simulink model "SensingSubsystem"  (R2026a)
settings: Solver=ode15s  StopTime=10  FixedStep=1e-3  MaxStep=1e-6  RelTol=1e-5
model workspace (MAT data in the model file):
  SL_ROS_VariableLengthArrays_MaxSizes.CommonInfo.ArrayTruncateAction = 'EmitWarning'
  SL_ROS_VariableLengthArrays_MaxSizes.MsgTypeMap = containers.Map
  SL_ROS_VariableLengthArrays_MaxSizes.MsgTypeMap.serialization.keys = {'sensor_msgs/Image'}
  SL_ROS_VariableLengthArrays_MaxSizes.MsgTypeMap.serialization.values{1}(1).PropertyName = 'data'
  SL_ROS_VariableLengthArrays_MaxSizes.MsgTypeMap.serialization.values{1}(1).DataType = 'uint8'
  SL_ROS_VariableLengthArrays_MaxSizes.MsgTypeMap.serialization.values{1}(1).MaxLength = 512
  SL_ROS_VariableLengthArrays_MaxSizes.MsgTypeMap.serialization.values{1}(2).PropertyName = 'encoding'
  SL_ROS_VariableLengthArrays_MaxSizes.MsgTypeMap.serialization.values{1}(2).DataType = 'uint8'
  SL_ROS_VariableLengthArrays_MaxSizes.MsgTypeMap.serialization.values{1}(2).MaxLength = 128
  SL_ROS_VariableLengthArrays_MaxSizes.MsgTypeMap.serialization.uniformity = 0
  SL_ROS_VariableLengthArrays_MaxSizes.MsgTypeMap.serialization.keyType = 'char'
  SL_ROS_VariableLengthArrays_MaxSizes.MsgTypeMap.serialization.valueType = 'any'
undefined symbols (not defined in the file or in its folder): AS7341_8Channel, BPW34_Photodiode, DS18B20_Temperature, MS5837_Pressure, sandy_sensors
libraries: fl_lib x32, nesl_utility x22, ee_lib x6, ros2lib x4
(part 1 of 2)
settings Model: Creator=skips  LastModifiedBy=skips
settings HardwareCC: ProdBitPerLong=64.0  ProdHWDeviceType=Intel->x86-64 (Linux 64)  UseEmbeddedCoderFeatures=off
settings RTWCC: SystemTargetFile=ert.tlc  HardwareBoard=Robot Operating System 2 (ROS 2)  TLCOptions="-aInlineSetEventsForThisBaseRateFcn=TLC_FALSE -aSuppressMultiTaskScheduler=TLC_FALSE  -aRateBasedStepFcn=0"  Toolchain=Colcon Tools  TargetLang=C++  Description=Embedded Coder
settings ERTTargetCC: ExtModeTransport=2.0  ExtModeAutomaticAllocSize=off  RootIOFormat=Structure reference  CodeInterfacePackaging=C++ class  SupportNonInlinedSFcns=on

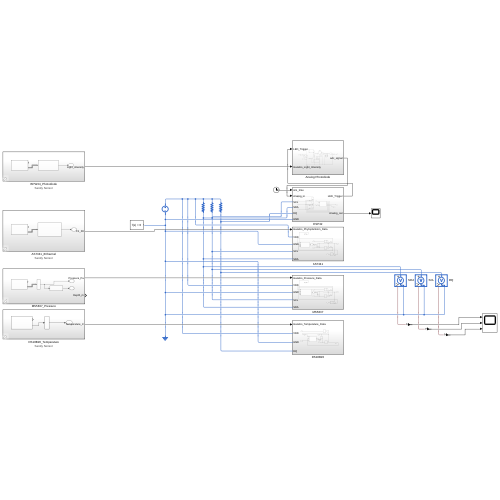
[thumbnail: Simulink's stored preview of the top-level diagram]
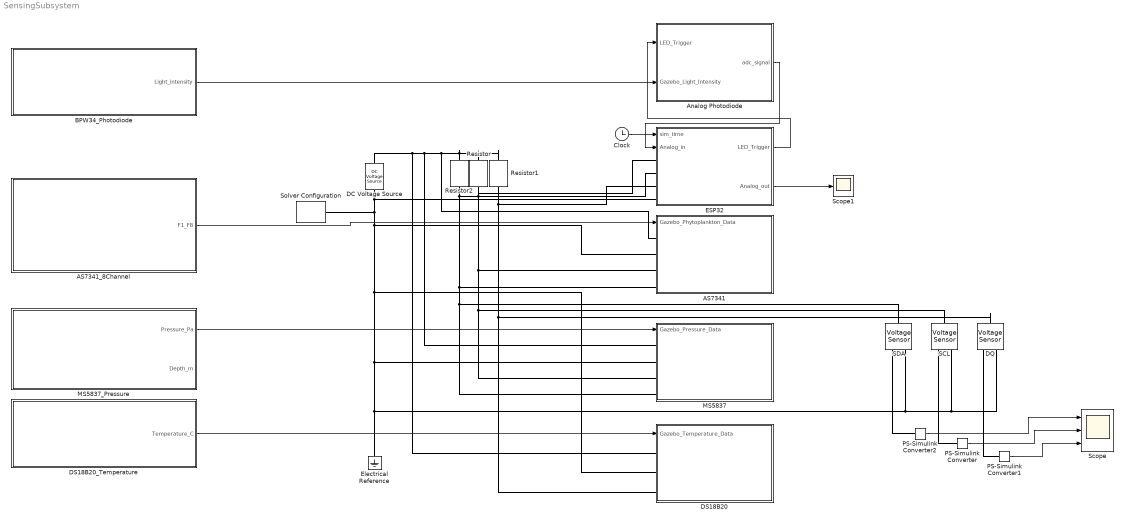
== system SensingSubsystem ==
  AS7341 : Subsystem
  AS7341_8Channel : Subsystem  Description=AS7341 8-channel proxy. Subscribes to /sandy/as7341_down (sensor_msgs/Image, 8x8 RGB from Gazebo) and synthesises 8 spectral channels F1..F8 (415, 445, 480, 515, 555, 590, 630, 680 nm). Output is uint16(1x8), matching the AS7341 16-bit ADC range. NOTE: This is a synthesis from broadband RGB. Useful for testing detection logic and data pipelines; not physically accurate for spectral retrieval algorithms.  AncestorBlock=sandy_sensors/AS7341_8Channel
      settings: AttributesFormatString=Sandy Sensor
  Analog Photodiode : Subsystem
  BPW34_Photodiode : Subsystem  Description=BPW34 photodiode proxy. Subscribes to /sandy/photodiode_side (sensor_msgs/Image, 4x4 RGB from Gazebo) and outputs a scalar irradiance in [0, 1]. Multiply by your photocurrent scale factor (e.g. 5e-7 A) before feeding into the TIA.  AncestorBlock=sandy_sensors/BPW34_Photodiode
      settings: AttributesFormatString=Sandy Sensor
  Clock : Clock
  DC Voltage Source : ee_lib/Additional Components/SPICE Sources/DC Voltage Source  DC=3.3 V
  DQ : fl_lib/Electrical/Electrical Sensors/Voltage Sensor
  DS18B20 : Subsystem
  DS18B20_Temperature : Subsystem  Description=DS18B20 temperature proxy. Subscribes to /sandy/temperature (sensor_msgs/Temperature, published by the helper node from the Antarctic depth profile OR a manual slider). Outputs scalar T in C.  AncestorBlock=sandy_sensors/DS18B20_Temperature
      settings: AttributesFormatString=Sandy Sensor
  ESP32 : Subsystem
  Electrical Reference : fl_lib/Electrical/Electrical Elements/Electrical Reference
  MS5837 : Subsystem
  MS5837_Pressure : Subsystem  Description=MS5837-30BA proxy. Subscribes to /sandy/pressure (sensor_msgs/FluidPressure, computed from buoy Z by the helper node). Outputs absolute pressure in Pa AND depth in m (depth = (P - 101325) / (1028 * 9.80665)).  AncestorBlock=sandy_sensors/MS5837_Pressure
      settings: AttributesFormatString=Sandy Sensor
  PS-Simulink Converter : nesl_utility/PS-Simulink Converter  PhysicalDomain=network_engine_domain  SubClassName=ps_output  LeftPortType=input  RightPortType=output  PseudoPeriodic=off  Frequencies=[]  VectorFormat=inherit  Unit=inherit  AffineConversion=off
  PS-Simulink Converter1 : nesl_utility/PS-Simulink Converter  PhysicalDomain=network_engine_domain  SubClassName=ps_output  LeftPortType=input  RightPortType=output  PseudoPeriodic=off  Frequencies=[]  VectorFormat=inherit  Unit=inherit  AffineConversion=off
  PS-Simulink Converter2 : nesl_utility/PS-Simulink Converter  PhysicalDomain=network_engine_domain  SubClassName=ps_output  LeftPortType=input  RightPortType=output  PseudoPeriodic=off  Frequencies=[]  VectorFormat=inherit  Unit=inherit  AffineConversion=off
  Resistor : fl_lib/Electrical/Electrical Elements/Resistor  R=4700 Ohm  i_specify=off  i_priority=None  i=0 A  i_nominal_specify=off  i_nominal_value=1  i_nominal_unit=A  v_specify=off  v_priority=None  v=0 V  v_nominal_specify=off  v_nominal_value=1  v_nominal_unit=V
  Resistor1 : fl_lib/Electrical/Electrical Elements/Resistor  R=4700 Ohm  i_specify=off  i_priority=None  i=0 A  i_nominal_specify=off  i_nominal_value=1  i_nominal_unit=A  v_specify=off  v_priority=None  v=0 V  v_nominal_specify=off  v_nominal_value=1  v_nominal_unit=V
  Resistor2 : fl_lib/Electrical/Electrical Elements/Resistor  R=4700 Ohm  i_specify=off  i_priority=None  i=0 A  i_nominal_specify=off  i_nominal_value=1  i_nominal_unit=A  v_specify=off  v_priority=None  v=0 V  v_nominal_specify=off  v_nominal_value=1  v_nominal_unit=V
  SCL : fl_lib/Electrical/Electrical Sensors/Voltage Sensor
  SDA : fl_lib/Electrical/Electrical Sensors/Voltage Sensor
  Scope : Scope  NumInputPorts=3
      settings: ActiveDisplayYMinimum=3.1434378707500259  ActiveDisplayYMaximum=3.3880168227126775
  Scope1 : Scope
      settings: ActiveDisplayYMinimum=-121086.7377727352  ActiveDisplayYMaximum=114154.80125551928
  Solver Configuration : nesl_utility/Solver Configuration  PhysicalDomain=network_engine_domain  SubClassName=solver  LeftPortType=input  RightPortType=generic  Tones=[]  Harmonics=[]  SimulateNoise=off  Profile=off  UseLocalSampling=off  EnableSwitchedLinearOptims=on  FrequencyDomain=off  UseCCode=off  RelTol=0.001  AbsTol=0.001  MinStep=1e-09  ToWorkspace=off  RevertToSquareIcSolve=off  NumHomotopyIterations=100  PhasorMode=off  PhasorModeNumHarmonics=1  ConsistencySolver=NEWTON_XTOL_AFTER_FTOL  CanonicalOrdering=CANONICAL  OptimizeIntermediates=OPTIMIZED  IndexReductionMethod=DerivativeReplacement  DoDC=off  ResidualTolerance=1e-09  ConsistencyTolSource=GLOBAL  ConsistencyAbsTol=0.001  ConsistencyRelTol=0.001  ConsistencyTolFactor=0.001  UseLocalSolver=off  LocalSolverChoice=NE_BACKWARD_EULER_ADVANCER  ResolveIndetEquations=on  FunctionEvalNumThread=1  LocalSolverSampleTime=0.001  DoFixedCost=off  MaxNonlinIter=3  MaxModeIter=2  ComputeImpulses=off  ImpulseIterations=2  LinearAlgebra=auto  LinearAlgebraNumThread=0  EquationFormulation=NE_TIME_EF  DelaysMemoryBudget=1024  AutomaticFiltering=on  FilteringTimeConstant=0.001  PartitionStorageMethod=AS_NEEDED  PartitionMemoryBudget=1024  PartitionMethod=ROBUST  MultibodyUseLocalSolver=off  MultibodyLocalSolverChoice=ODE1  MultibodyLocalSolverSampleTime=0.001
  wires:
  Clock/1 -> ESP32/1(sim_time)
  PS-Simulink Converter2/1 -> Scope/1
  PS-Simulink Converter/1 -> Scope/2
  PS-Simulink Converter1/1 -> Scope/3
  AS7341_8Channel/1(F1_F8) -> AS7341/1(Gazebo_Phytoplankton_Data)
  DS18B20_Temperature/1(Temperature_C) -> DS18B20/1(Gazebo_Temperature_Data)
  Analog Photodiode/1(adc_signal) -> ESP32/2(Analog_in)
  ESP32/1(LED_Trigger) -> Analog Photodiode/1(LED_Trigger)
  ESP32/2(Analog_out) -> Scope1/1
  BPW34_Photodiode/1(Light_intensity) -> Analog Photodiode/2(Gazebo_Light_Intensity)
  MS5837_Pressure/1(Pressure_Pa) -> MS5837/1(Gazebo_Pressure_Data)
  connections:
  Electrical Reference/LConn1 -- SDA/RConn2 -- DQ/RConn2 -- SCL/RConn2 -- ESP32/LConn4 -- DC Voltage Source/RConn1 -- Solver Configuration/RConn1 -- AS7341/LConn2 -- DS18B20/LConn2 -- MS5837/LConn2
  Resistor/LConn1 -- AS7341/LConn1 -- MS5837/LConn1 -- DS18B20/LConn1 -- DC Voltage Source/LConn1 -- Resistor2/LConn1 -- Resistor1/LConn1
  Resistor1/RConn1 -- DQ/LConn1 -- DS18B20/LConn3 -- ESP32/LConn3
  Resistor/RConn1 -- SCL/LConn1 -- MS5837/LConn3 -- AS7341/LConn3 -- ESP32/LConn1
  Resistor2/RConn1 -- ESP32/LConn2 -- SDA/LConn1 -- MS5837/LConn4 -- AS7341/LConn4
  SDA/RConn1 -- PS-Simulink Converter2/LConn1
  SCL/RConn1 -- PS-Simulink Converter/LConn1
  DQ/RConn1 -- PS-Simulink Converter1/LConn1

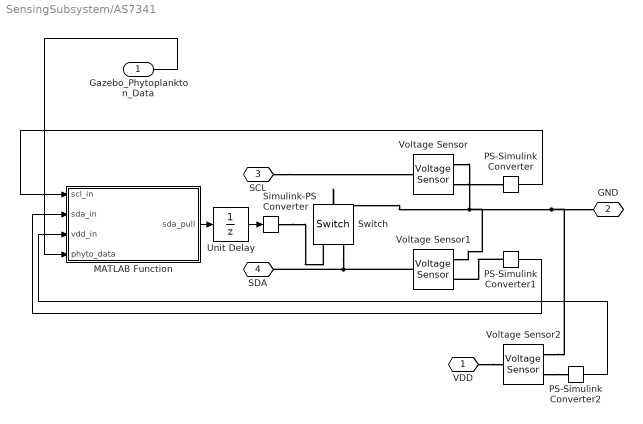
== system SensingSubsystem/AS7341 ==
  Gazebo_Phytoplankton_Data : Inport
  MATLAB Function : MATLAB Function  TreatAsAtomicUnit=on  SystemSampleTime=1e-3
  PS-Simulink Converter : nesl_utility/PS-Simulink Converter  PhysicalDomain=network_engine_domain  SubClassName=ps_output  LeftPortType=input  RightPortType=output  PseudoPeriodic=off  Frequencies=[]  VectorFormat=inherit  Unit=inherit  AffineConversion=off
  PS-Simulink Converter1 : nesl_utility/PS-Simulink Converter  PhysicalDomain=network_engine_domain  SubClassName=ps_output  LeftPortType=input  RightPortType=output  PseudoPeriodic=off  Frequencies=[]  VectorFormat=inherit  Unit=inherit  AffineConversion=off
  PS-Simulink Converter2 : nesl_utility/PS-Simulink Converter  PhysicalDomain=network_engine_domain  SubClassName=ps_output  LeftPortType=input  RightPortType=output  PseudoPeriodic=off  Frequencies=[]  VectorFormat=inherit  Unit=inherit  AffineConversion=off
  Simulink-PS Converter : nesl_utility/Simulink-PS Converter  PhysicalDomain=network_engine_domain  SubClassName=ps_input  LeftPortType=input  RightPortType=output  PseudoPeriodic=off  Frequencies=[]  NoiseDistribution=none  NoiseParameters=[]  Unit=1  AffineConversion=off  FilteringAndDerivatives=provide  SimscapeFilterOrder=1  InputFilterTimeConstant=0.001  UdotUserProvided=0
  Switch : fl_lib/Electrical/Electrical Elements/Switch  R_closed=0.01 Ohm  G_open=1e-8 1/Ohm  Threshold=0.5  i_specify=off  i_priority=None  i=0 A  i_nominal_specify=off  i_nominal_value=1  i_nominal_unit=A  v_specify=off  v_priority=None  v=0 V  v_nominal_specify=off  v_nominal_value=1  v_nominal_unit=V
  Unit Delay : UnitDelay  SampleTime=-1
  Voltage Sensor : fl_lib/Electrical/Electrical Sensors/Voltage Sensor
  Voltage Sensor1 : fl_lib/Electrical/Electrical Sensors/Voltage Sensor
  Voltage Sensor2 : fl_lib/Electrical/Electrical Sensors/Voltage Sensor
  VDD : PMIOPort  Side=Left
  GND : PMIOPort  Port=2  Side=Left
  SCL : PMIOPort  Port=3  Side=Left
  SDA : PMIOPort  Port=4  Side=Left
  wires:
  PS-Simulink Converter1/1 -> MATLAB Function/2(sda_in)
  PS-Simulink Converter/1 -> MATLAB Function/1(scl_in)
  PS-Simulink Converter2/1 -> MATLAB Function/3(vdd_in)
  Gazebo_Phytoplankton_Data/1 -> MATLAB Function/4(phyto_data)
  Unit Delay/1 -> Simulink-PS Converter/1
  MATLAB Function/1(sda_pull) -> Unit Delay/1
  connections:
  SCL/RConn1 -- Voltage Sensor/LConn1
  Voltage Sensor/RConn2 -- Voltage Sensor1/RConn2 -- Voltage Sensor2/RConn2 -- GND/RConn1 -- Switch/LConn1
  Voltage Sensor1/LConn1 -- Switch/RConn2 -- SDA/RConn1
  Voltage Sensor/RConn1 -- PS-Simulink Converter/LConn1
  PS-Simulink Converter1/LConn1 -- Voltage Sensor1/RConn1
  Simulink-PS Converter/RConn1 -- Switch/RConn1
  VDD/RConn1 -- Voltage Sensor2/LConn1
  Voltage Sensor2/RConn1 -- PS-Simulink Converter2/LConn1

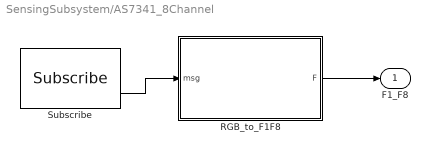
== system SensingSubsystem/AS7341_8Channel ==
  RGB_to_F1F8 : MATLAB Function  TreatAsAtomicUnit=on
  Subscribe : ros2lib/Subscribe  topicSource=Specify your own  topic=/sandy/as7341_down  messageType=sensor_msgs/Image  sampleTime=0.1  QOSHistory=Keep last  QOSDepth=5  QOSReliability=Best effort  QOSDurability=Volatile  QOSDeadline=Inf  QOSLifespan=Inf  QOSLiveliness=Automatic  QOSLeaseDuration=Inf  QOSAvoidROSNamespaceConventions=off
  F1_F8 : Outport
  wires:
  RGB_to_F1F8/1(F) -> F1_F8/1
  Subscribe/2 -> RGB_to_F1F8/1(msg)

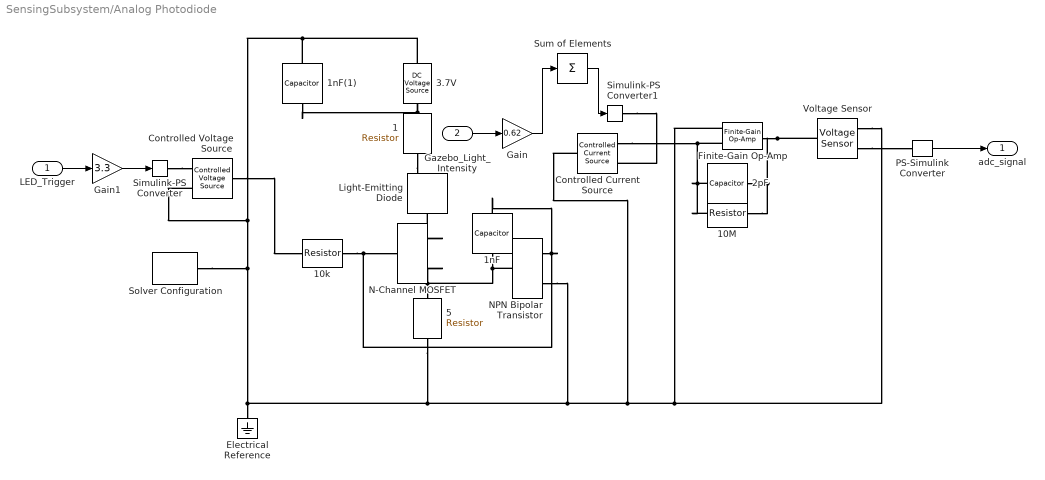
== system SensingSubsystem/Analog Photodiode ==
  LED_Trigger : Inport
  Gazebo_Light_Intensity : Inport  Port=2
  1 : fl_lib/Electrical/Electrical Elements/Resistor  R=1 Ohm  i_specify=off  i_priority=None  i=0 A  i_nominal_specify=off  i_nominal_value=1  i_nominal_unit=A  v_specify=off  v_priority=None  v=0 V  v_nominal_specify=off  v_nominal_value=1  v_nominal_unit=V
  10M : fl_lib/Electrical/Electrical Elements/Resistor  R=10 MOhm  i_specify=off  i_priority=None  i=0 A  i_nominal_specify=off  i_nominal_value=1  i_nominal_unit=A  v_specify=off  v_priority=None  v=0 V  v_nominal_specify=off  v_nominal_value=1  v_nominal_unit=V
  10k : fl_lib/Electrical/Electrical Elements/Resistor  R=10000 Ohm  i_specify=off  i_priority=None  i=0 A  i_nominal_specify=off  i_nominal_value=1  i_nominal_unit=A  v_specify=off  v_priority=None  v=0 V  v_nominal_specify=off  v_nominal_value=1  v_nominal_unit=V
  1nF : fl_lib/Electrical/Electrical Elements/Capacitor  c=2e-9 F  r=1e-6 Ohm  g=0 1/Ohm  i_specify=off  i_priority=None  i=0 A  i_nominal_specify=off  i_nominal_value=1  i_nominal_unit=A  v_specify=off  v_priority=None  v=0 V  v_nominal_specify=off  v_nominal_value=1  v_nominal_unit=V  vc_specify=off  vc_priority=High  vc=0 V  vc_nominal_specify=off  vc_nominal_value=1  vc_nominal_unit=V
  1nF(1) : fl_lib/Electrical/Electrical Elements/Capacitor  c=1 nF  r=1e-6 Ohm  g=0 1/Ohm  i_specify=off  i_priority=None  i=0 A  i_nominal_specify=off  i_nominal_value=1  i_nominal_unit=A  v_specify=off  v_priority=None  v=0 V  v_nominal_specify=off  v_nominal_value=1  v_nominal_unit=V  vc_specify=off  vc_priority=High  vc=0 V  vc_nominal_specify=off  vc_nominal_value=1  vc_nominal_unit=V
  2pF : fl_lib/Electrical/Electrical Elements/Capacitor  c=2 pF  r=1e-6 Ohm  g=0 1/Ohm  i_specify=off  i_priority=None  i=0 A  i_nominal_specify=off  i_nominal_value=1  i_nominal_unit=A  v_specify=off  v_priority=None  v=0 V  v_nominal_specify=off  v_nominal_value=1  v_nominal_unit=V  vc_specify=off  vc_priority=High  vc=0 V  vc_nominal_specify=off  vc_nominal_value=1  vc_nominal_unit=V
  3.7V : ee_lib/Additional Components/SPICE Sources/DC Voltage Source  DC=3.7 V
  5 : fl_lib/Electrical/Electrical Elements/Resistor  R=5 Ohm  i_specify=off  i_priority=None  i=0 A  i_nominal_specify=off  i_nominal_value=1  i_nominal_unit=A  v_specify=off  v_priority=None  v=0 V  v_nominal_specify=off  v_nominal_value=1  v_nominal_unit=V
  Controlled Current Source : fl_lib/Electrical/Electrical Sources/Controlled Current Source
  Controlled Voltage Source : fl_lib/Electrical/Electrical Sources/Controlled Voltage Source
  Electrical Reference : fl_lib/Electrical/Electrical Elements/Electrical Reference
  Finite-Gain Op-Amp : ee_lib/Integrated Circuits/Finite-Gain Op-Amp  A=1e5  Rin=1e12 Ohm  Rout=10 Ohm  Vmin=0.02 V  Vmax=3.3 V  noise_mode=ee.enum.mode.enabled  v_noise=30e-9 V/Hz^(1/2)  noise_prm=ee.enum.ic.noiseParameterization.same  i_noise=0.6e-15 A/Hz^(1/2)  ip_noise=0.5e-12 A/Hz^(1/2)  in_noise=0.5e-12 A/Hz^(1/2)  sample_time=1e-3 s  repeatability=ee.enum.ic.repeatability.notRepeatable  auto_seed_v=3890346746  auto_seed_ip=545404223  auto_seed_in=3922919431  user_seed_v=0  user_seed_ip=0  user_seed_in=0
  Gain : Gain  Gain=0.62  OutDataTypeStr=Inherit: Same as input
  Gain1 : Gain  Gain=3.3
  Light-Emitting Diode : ee_lib/Sensors & Transducers/Light-Emitting Diode  Gain=0.005 W/A  prmExp=ee.enum.diode.led.useTwo  I12=[.0017, .003] A  V12=[.9, 1.05] V  IS=5e-5 A  ec=10  RS=0.1 Ohm  Tmeas=25 degC  C_param=ee.enum.diode.capParam.fixed  CJ=20 pF  CJ0=20 pF  Vvec=[.1, 10, 100] V  Cvec=[15, 10, 2] pF  VJ=1 V  Mgrad=0.5  FC=0.5  T_param=ee.enum.diode.temperatureParam.off  Tdevice=25 degC  IS_T2=1.8e-4 A  I1_T2=0.0034 A  V1_T2=1.05 V  Tmeas2=125 degC  EG_param=ee.enum.diode.egapParam.material_si  EG=1.11 eV  XTI_param=ee.enum.diode.xtiParam.pn  XTI=3  i_specify=off  i_priority=None  i=0 A  i_nominal_specify=off  i_nominal_value=1  i_nominal_unit=A  v_specify=off  v_priority=None  v=0 V  v_nominal_specify=off  v_nominal_value=1  v_nominal_unit=V  v_capacitor_specify=off  v_capacitor_priority=None  v_capacitor=0 V  v_capacitor_nominal_specify=off  v_capacitor_nominal_value=1  v_capacitor_nominal_unit=V  Qj_specify=off  Qj_priority=High  Qj=0 C  Qj_nominal_specify=off  Qj_nominal_value=1  Qj_nominal_unit=C  thermal_network_parameterization=ee.enum.thermalNetworkTopology.junctionCase  Rth=[0, 10] K/W  Rth_Cauer=[1, 3, 10] K/W  Rth_Foster=[.08, .14, .22, .16] K/W  thermal_mass_parameterization=ee.enum.thermalNetwork.timeconstant  thermal_mass=[0, 1] J/K  thermal_mass_Cauer=[1.5, 2, 3] J/K  thermal_mass_Foster=[.001, .005, .05, .5] J/K  thermal_time_constant=[0, 10] s  thermal_time_constant_Cauer=[1, 3, 10] s  thermal_time_constant_Foster=[7e-05, .0007, .01, .08] s  thermal_mass_initial_temperatures=[25, 25] degC  thermal_mass_initial_temperatures_Cauer=[25, 25, 25] degC  steadyState_Foster=simscape.enum.onoff.on  Tvec_initial_Foster=[25, 25, 25, 25] degC
  N-Channel MOSFET : ee_lib/Semiconductors & Converters/N-Channel MOSFET  paramTerminal=ee.enum.mosfet.numberOfTerminals.three  parameterization=ee.enum.mosfet.parameterization.datasheet  Beta=5.0 A/V^2  Rds=0.035 Ohm  Id=16 A  Vgs=5 V  Vth=2.1 V  Vth0=1.7 V  lam=0 1/V  gamma_vth=0.5 V^(1/2)  phib=0.5 V  Vth1=1.9071 V  Vbs1=-1 V  Vth2=2.066 V  Vbs2=-2 V  Tmeas=0 degC  Vgs_vec=[-1, -.5, 2, 3, 4, 5] V  Vds_vec=[0, 2, 4, 8, 12, 16, 20] V  Vbs_vec=[0, -4, -6, -12] V  T_vec=[25, 125] degC  Vth_vec=[.4, 1.2, 1.4, 1.45] V  Vth_mat=[.4, .35; 1.2, 1.15; 1.4, 1.35; 1.45, 1.4] V  Ids_mat=[0, 0, 0, 0, 0, 0, 0; 0, 0, 0, 0, 0, 0, 0; 0, .003, .0038, .0043, .0046, .0048, .0049; 0, .0055, .008, .009, .0095, .01, .0101; 0, .0115, .016, .018, .019, .0195, .02; 0, .0152, .0225, .0265, .028, .0295, .03] A  Ids_mat0=[0, 0, 0, 0, 0, 0, 0; 0, 0, 0, 0, 0, 0, 0; 0, .003, .0038, .0043, .0046, .0048, .0049; 0, .0055, .008, .009, .0095, .01, .0101; 0, .0115, .016, .018, .019, .0195, .02; 0, .0152, .0225, .0265, .028, .0295, .03] A  Ids_mat_3D=zeros(6, 7, 2) A  Ids_mat_3D0=zeros(6, 7, 2) A  IV_table_symmetry=ee.enum.mosfet.symmetricNIV.no  RS=0.0001 Ohm  RD=0.01 Ohm  RB=0.001 Ohm  LeadRs=0 Ohm  LeadRd=0 Ohm  LeadRg=0 Ohm  LeadRb=0 Ohm  LS=0 nH  LD=0 nH  LG=0 nH  LB=0 nH  C_param=ee.enum.mosfet.capacitanceParam.fixedciss  C_GS=270 pF  C_GD=80 pF  C_GB=0 pF  C_DS=0 pF  C_iss=1000 pF  C_rss=120 pF  C_oss=0 pF  C_iss_vec=[720, 700, 590, 470, 390, 310] pF  C_rss_vec=[450, 400, 300, 190, 95, 55] pF  C_oss_vec=[900, 810, 690, 420, 270, 170] pF  C_GS_vec=[270, 300, 290, 280, 295, 255] pF  C_GD_vec=[450, 400, 300, 190, 95, 55] pF  C_GB_vec=[270, 300, 290, 280, 295, 255] pF  C_Vgs_vec=0 V  C_DS_vec=[450, 410, 390, 230, 175, 115] pF  C_Vds_vec=[.1, .3, 1, 3, 10, 30] V  V_GS_for_cap_data=0 V  charge_linearity_param=ee.enum.mosfet.cgdLinearity.constant  C_OX=200 pF  V_C_OX=-0.5 V  charge_linearity_param_vgb=ee.enum.mosfet.cgbLinearity.instantly  charge_linearity_param_with_vgb=ee.enum.mosfet.cgbLinearityWithSeparateCgb.instantly  Di_param=ee.enum.mosfet.diodeParam.no  IsDiode=1e-12 A  Vbi=0.6 V  n=1  Cj0Diode=0 pF  TT=50e-9 s  Tmeas_dio=25 degC  TableTypeNoT=ee.enum.mosfet.tableType.IfMat  TableType=ee.enum.diode.tableType.IfMat  IfVec=[.07, .12, .19, 1.75, 4.24, 7.32, 11.2] A  IfMat=[.07, .12, .19, 1.75, 4.24, 7.32, 11.2; .16, .3, .72, 2.14, 4.02, 6.35, 9.12] A  VfVecV=[.9, 1.15, 1.25, 1.5, 1.75, 2.17, 2.6, 2.85] V  VfMatV=[.9, 1.15, 1.25, 1.5, 1.75, 2.17, 2.6, 2.85; .58, .68, .75, 1.1, 1.38, 1.77, 2.27, 2.7] V  TjVec=[25, 125] degC  VfVec=[.5, .7, .9, 1.3, 1.7, 2.1, 2.5] V  IfVecV=[.1, .2, .5, 1, 2, 4, 7, 10] A  diode_Goff=1e-12 1/Ohm  prmDatasheet=ee.enum.temperatureParameterization.none  prmEquCoeff=ee.enum.temperatureParameterization.none  dVth_dT=-6 mV/K  dVth0_dT=-6 mV/K  Rds_T2=0.037 Ohm  BEXDatasheet=-1.5  BEXEquCoeff=-1.5  etaisDatasheet=3  etaisEquCoeff=3  Tmeas2=125 degC  etaisTabulated=3  TdeviceDatasheet=25 degC  TdeviceEquCoeff=25 degC  TdeviceTabulated=25 degC  i_g_specify=off  i_g_priority=None  i_g=0 A  i_g_nominal_specify=off  i_g_nominal_value=1  i_g_nominal_unit=A  i_d_specify=off  i_d_priority=None  i_d=0 A  i_d_nominal_specify=off  i_d_nominal_value=1  i_d_nominal_unit=A  i_b_specify=off  i_b_priority=None  i_b=0 A  i_b_nominal_specify=off  i_b_nominal_value=1  i_b_nominal_unit=A  voltage_gs_specify=off  voltage_gs_priority=None  voltage_gs=0 V  voltage_gs_nominal_specify=off  voltage_gs_nominal_value=1  voltage_gs_nominal_unit=V  voltage_ds_specify=off  voltage_ds_priority=None  voltage_ds=0 V  voltage_ds_nominal_specify=off  voltage_ds_nominal_value=1  voltage_ds_nominal_unit=V  voltage_bs_specify=off  voltage_bs_priority=None  voltage_bs=0 V  voltage_bs_nominal_specify=off  voltage_bs_nominal_value=1  voltage_bs_nominal_unit=V  v_Cgs_specify=off  v_Cgs_priority=High  v_Cgs=0 V  v_Cgs_nominal_specify=off  v_Cgs_nominal_value=1  v_Cgs_nominal_unit=V  v_Cds_specify=off  v_Cds_priority=High  v_Cds=0 V  v_Cds_nominal_specify=off  v_Cds_nominal_value=1  v_Cds_nominal_unit=V  v_Cbs_specify=off  v_Cbs_priority=High  v_Cbs=0 V  v_Cbs_nominal_specify=off  v_Cbs_nominal_value=1  v_Cbs_nominal_unit=V  thermal_network_parameterization=ee.enum.thermalNetworkTopology.junctionCase  Rth=[0, 10] K/W  Rth_Cauer=[1, 3, 10] K/W  Rth_Foster=[.08, .14, .22, .16] K/W  thermal_mass_parameterization=ee.enum.thermalNetwork.timeconstant  thermal_mass=[0, 1] J/K  thermal_mass_Cauer=[.1, .3, 1] J/K  thermal_mass_Foster=[.001, .005, .05, .5] J/K  thermal_time_constant=[0, 10] s  thermal_time_constant_Cauer=[1, 3, 10] s  thermal_time_constant_Foster=[7e-05, .0007, .01, .08] s  thermal_mass_initial_temperatures=[25, 25] degC  thermal_mass_initial_temperatures_Cauer=[25, 25, 25] degC  Tvec_initial_Foster=[25, 25, 25, 25] degC  betaref=18 A/V^2  Vfbref=-1.1 V  gamma=3.5 V^(1/2)  phib2ref=1 V  thesatref=0.4 1/V  alpha=0  Vp=5e-2 V  thesrref=0 1/V  m=8  Tref=25 degC  Rsref=2e-3 Ohm  Rdref=0.17 Ohm  Rgref=8.4 Ohm  Rbref=2e-3 Ohm  Cox=1500 pF  Cgso=100 pF  Cgdo=14 pF  Isref=5.2e-13 A  Cj0=480 pF  Tprm=ee.enum.temperatureParameterization.none  etabet=1.3  Stvfb=5e-4 V/K  Stphib=-8.5e-4 V/K  etasat=1.04  etasr=0.65  etar=0.95  etais=3  Tsim=25 degC  Ig_specify=off  Ig_priority=None  Ig=0 A  Ig_nominal_specify=off  Ig_nominal_value=1  Ig_nominal_unit=nA  Ids_specify=off  Ids_priority=None  Ids=0 A  Ids_nominal_specify=off  Ids_nominal_value=1  Ids_nominal_unit=A  Ib_specify=off  Ib_priority=None  Ib=0 A  Ib_nominal_specify=off  Ib_nominal_value=1  Ib_nominal_unit=uA  V_gs_specify=off  V_gs_priority=None  V_gs=0 V  V_gs_nominal_specify=off  V_gs_nominal_value=1  V_gs_nominal_unit=V  V_ds_specify=off  V_ds_priority=None  V_ds=0 V  V_ds_nominal_specify=off  V_ds_nominal_value=1  V_ds_nominal_unit=V  V_bs_specify=off  V_bs_priority=None  V_bs=0 V  V_bs_nominal_specify=off  V_bs_nominal_value=1  V_bs_nominal_unit=V  QGoverCox_specify=off  QGoverCox_priority=None  QGoverCox=0 V  QGoverCox_nominal_specify=off  QGoverCox_nominal_value=1  QGoverCox_nominal_unit=V  QDoverCox_specify=off  QDoverCox_priority=None  QDoverCox=0 V  QDoverCox_nominal_specify=off  QDoverCox_nominal_value=1  QDoverCox_nominal_unit=V  QBoverCox_specify=off  QBoverCox_priority=None  QBoverCox=0 V  QBoverCox_nominal_specify=off  QBoverCox_nominal_value=1  QBoverCox_nominal_unit=V  T0=[25, 25] degC  T0_Cauer=[25, 25, 25] degC
  NPN Bipolar Transistor : ee_lib/Semiconductors & Converters/NPN Bipolar Transistor  parameterization=1  BF=100  IS=1e-14 A  VAF=200 V  hfe=300  hoe=50e-6 1/Ohm  Ic_h=1 mA  Vce_h=5 V  V1=0.65 V  I1=0.5 mA  BR=1  Tmeas=0 degC  RC=0.01 Ohm  RE=1e-4 Ohm  RB=1 Ohm  C_BC=5 pF  C_BE=5 pF  TF=0 us  TR=0 us  prmDatasheet=1  prmEquCoeff=1  hfe_T2=125  XTB=0  V1_T2=0.45 V  I1_T2=0.5 mA  Tmeas2=125 degC  EG=1.11 eV  XTI=3  TdeviceDatasheet=25 degC  TdeviceEquCoeff=25 degC  ec=1  ib_specify=off  ib_priority=None  ib=0 A  ib_nominal_specify=off  ib_nominal_value=1  ib_nominal_unit=A  ic_specify=off  ic_priority=None  ic=0 A  ic_nominal_specify=off  ic_nominal_value=1  ic_nominal_unit=A  vce_specify=off  vce_priority=None  vce=0 V  vce_nominal_specify=off  vce_nominal_value=1  vce_nominal_unit=V  vbe_specify=off  vbe_priority=None  vbe=0 V  vbe_nominal_specify=off  vbe_nominal_value=1  vbe_nominal_unit=V  Qbc_specify=off  Qbc_priority=High  Qbc=0 C  Qbc_nominal_specify=off  Qbc_nominal_value=1  Qbc_nominal_unit=uC  Qbe_specify=off  Qbe_priority=High  Qbe=0 C  Qbe_nominal_specify=off  Qbe_nominal_value=1  Qbe_nominal_unit=uC  thermal_network_parameterization=ee.enum.thermalNetworkTopology.junctionCase  Rth=[0, 10] K/W  Rth_Cauer=[1, 3, 10] K/W  Rth_Foster=[.08, .14, .22, .16] K/W  thermal_mass_parameterization=ee.enum.thermalNetwork.timeconstant  thermal_mass=[0, 1] J/K  thermal_mass_Cauer=[.1, .3, 1] J/K  thermal_mass_Foster=[.001, .005, .05, .5] J/K  thermal_time_constant=[0, 10] s  thermal_time_constant_Cauer=[1, 3, 10] s  thermal_time_constant_Foster=[7e-05, .0007, .01, .08] s  thermal_mass_initial_temperatures=[25, 25] degC  thermal_mass_initial_temperatures_Cauer=[25, 25, 25] degC  Tvec_initial_Foster=[25, 25, 25, 25] degC
  PS-Simulink Converter : nesl_utility/PS-Simulink Converter  PhysicalDomain=network_engine_domain  SubClassName=ps_output  LeftPortType=input  RightPortType=output  PseudoPeriodic=off  Frequencies=[]  VectorFormat=inherit  Unit=V  AffineConversion=off
  Simulink-PS Converter : nesl_utility/Simulink-PS Converter  PhysicalDomain=network_engine_domain  SubClassName=ps_input  LeftPortType=input  RightPortType=output  PseudoPeriodic=off  Frequencies=[]  NoiseDistribution=none  NoiseParameters=[]  Unit=V  AffineConversion=off  FilteringAndDerivatives=zero  SimscapeFilterOrder=1  InputFilterTimeConstant=1e-7  UdotUserProvided=0
  Simulink-PS Converter1 : nesl_utility/Simulink-PS Converter  PhysicalDomain=network_engine_domain  SubClassName=ps_input  LeftPortType=input  RightPortType=output  PseudoPeriodic=off  Frequencies=[]  NoiseDistribution=none  NoiseParameters=[]  Unit=A  AffineConversion=off  FilteringAndDerivatives=provide  SimscapeFilterOrder=1  InputFilterTimeConstant=0.001  UdotUserProvided=0
  Solver Configuration : nesl_utility/Solver Configuration  PhysicalDomain=network_engine_domain  SubClassName=solver  LeftPortType=input  RightPortType=generic  Tones=[]  Harmonics=[]  SimulateNoise=off  Profile=off  UseLocalSampling=off  EnableSwitchedLinearOptims=on  FrequencyDomain=off  UseCCode=off  RelTol=0.001  AbsTol=0.001  MinStep=1e-09  ToWorkspace=off  RevertToSquareIcSolve=off  NumHomotopyIterations=100  PhasorMode=off  PhasorModeNumHarmonics=1  ConsistencySolver=NEWTON_XTOL_AFTER_FTOL  CanonicalOrdering=CANONICAL  OptimizeIntermediates=OPTIMIZED  IndexReductionMethod=DerivativeReplacement  DoDC=off  ResidualTolerance=1e-09  ConsistencyTolSource=GLOBAL  ConsistencyAbsTol=0.001  ConsistencyRelTol=0.001  ConsistencyTolFactor=0.001  UseLocalSolver=off  LocalSolverChoice=NE_BACKWARD_EULER_ADVANCER  ResolveIndetEquations=on  FunctionEvalNumThread=1  LocalSolverSampleTime=0.001  DoFixedCost=off  MaxNonlinIter=3  MaxModeIter=2  ComputeImpulses=off  ImpulseIterations=2  LinearAlgebra=auto  LinearAlgebraNumThread=0  EquationFormulation=NE_TIME_EF  DelaysMemoryBudget=1024  AutomaticFiltering=on  FilteringTimeConstant=0.001  PartitionStorageMethod=AS_NEEDED  PartitionMemoryBudget=1024  PartitionMethod=ROBUST  MultibodyUseLocalSolver=off  MultibodyLocalSolverChoice=ODE1  MultibodyLocalSolverSampleTime=0.001
  Sum of Elements : Sum  Inputs=+
  Voltage Sensor : fl_lib/Electrical/Electrical Sensors/Voltage Sensor
  adc_signal : Outport
  wires:
  Gazebo_Light_Intensity/1 -> Gain/1
  Gain/1 -> Sum of Elements/1
  Gain1/1 -> Simulink-PS Converter/1
  LED_Trigger/1 -> Gain1/1
  PS-Simulink Converter/1 -> adc_signal/1
  Sum of Elements/1 -> Simulink-PS Converter1/1
  connections:
  3.7V/RConn1 -- 1nF(1)/RConn1 -- Solver Configuration/RConn1 -- Controlled Current Source/LConn1 -- Finite-Gain Op-Amp/LConn1 -- Voltage Sensor/RConn2 -- NPN Bipolar Transistor/RConn2 -- 5/RConn1 -- Electrical Reference/LConn1 -- Controlled Voltage Source/RConn2
  1/LConn1 -- 1nF(1)/LConn1 -- 3.7V/LConn1
  1/RConn1 -- Light-Emitting Diode/LConn2
  N-Channel MOSFET/RConn1 -- Light-Emitting Diode/RConn1
  10k/RConn1 -- 1nF/LConn1 -- NPN Bipolar Transistor/RConn1 -- N-Channel MOSFET/LConn1
  N-Channel MOSFET/RConn2 -- NPN Bipolar Transistor/LConn1 -- 1nF/RConn1 -- 5/LConn1
  Simulink-PS Converter1/RConn1 -- Controlled Current Source/RConn1
  2pF/LConn1 -- Finite-Gain Op-Amp/LConn2 -- Controlled Current Source/RConn2 -- 10M/LConn1
  2pF/RConn1 -- Finite-Gain Op-Amp/RConn1 -- Voltage Sensor/LConn1 -- 10M/RConn1
  Simulink-PS Converter/RConn1 -- Controlled Voltage Source/RConn1
  Controlled Voltage Source/LConn1 -- 10k/LConn1
  Voltage Sensor/RConn1 -- PS-Simulink Converter/LConn1

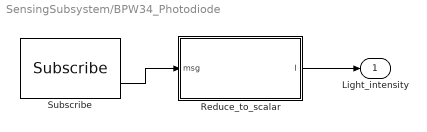
== system SensingSubsystem/BPW34_Photodiode ==
  Reduce_to_scalar : MATLAB Function  TreatAsAtomicUnit=on
  Subscribe : ros2lib/Subscribe  topicSource=Specify your own  topic=/sandy/photodiode_side  messageType=sensor_msgs/Image  sampleTime=0.1  QOSHistory=Keep last  QOSDepth=5  QOSReliability=Best effort  QOSDurability=Volatile  QOSDeadline=Inf  QOSLifespan=Inf  QOSLiveliness=Automatic  QOSLeaseDuration=Inf  QOSAvoidROSNamespaceConventions=off
  Light_intensity : Outport
  wires:
  Reduce_to_scalar/1(I) -> Light_intensity/1
  Subscribe/2 -> Reduce_to_scalar/1(msg)

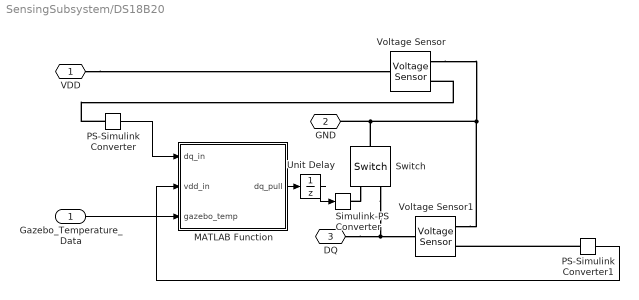
== system SensingSubsystem/DS18B20 ==
  Gazebo_Temperature_Data : Inport
  MATLAB Function : MATLAB Function  TreatAsAtomicUnit=on  SystemSampleTime=1e-3
  PS-Simulink Converter : nesl_utility/PS-Simulink Converter  PhysicalDomain=network_engine_domain  SubClassName=ps_output  LeftPortType=input  RightPortType=output  PseudoPeriodic=off  Frequencies=[]  VectorFormat=inherit  Unit=inherit  AffineConversion=off
  PS-Simulink Converter1 : nesl_utility/PS-Simulink Converter  PhysicalDomain=network_engine_domain  SubClassName=ps_output  LeftPortType=input  RightPortType=output  PseudoPeriodic=off  Frequencies=[]  VectorFormat=inherit  Unit=inherit  AffineConversion=off
  Simulink-PS Converter : nesl_utility/Simulink-PS Converter  PhysicalDomain=network_engine_domain  SubClassName=ps_input  LeftPortType=input  RightPortType=output  PseudoPeriodic=off  Frequencies=[]  NoiseDistribution=none  NoiseParameters=[]  Unit=1  AffineConversion=off  FilteringAndDerivatives=provide  SimscapeFilterOrder=1  InputFilterTimeConstant=0.001  UdotUserProvided=0
  Switch : fl_lib/Electrical/Electrical Elements/Switch  R_closed=0.01 Ohm  G_open=1e-8 1/Ohm  Threshold=0.5  i_specify=off  i_priority=None  i=0 A  i_nominal_specify=off  i_nominal_value=1  i_nominal_unit=A  v_specify=off  v_priority=None  v=0 V  v_nominal_specify=off  v_nominal_value=1  v_nominal_unit=V
  Unit Delay : UnitDelay  SampleTime=-1
  Voltage Sensor : fl_lib/Electrical/Electrical Sensors/Voltage Sensor
  Voltage Sensor1 : fl_lib/Electrical/Electrical Sensors/Voltage Sensor
  VDD : PMIOPort  Side=Left
  GND : PMIOPort  Port=2  Side=Left
  DQ : PMIOPort  Port=3  Side=Left
  wires:
  Gazebo_Temperature_Data/1 -> MATLAB Function/3(gazebo_temp)
  PS-Simulink Converter/1 -> MATLAB Function/1(dq_in)
  PS-Simulink Converter1/1 -> MATLAB Function/2(vdd_in)
  MATLAB Function/1(dq_pull) -> Unit Delay/1
  Unit Delay/1 -> Simulink-PS Converter/1
  connections:
  VDD/RConn1 -- Voltage Sensor/LConn1
  Voltage Sensor/RConn2 -- Voltage Sensor1/RConn2 -- Switch/LConn1 -- GND/RConn1
  PS-Simulink Converter/LConn1 -- Voltage Sensor/RConn1
  DQ/RConn1 -- Switch/RConn2 -- Voltage Sensor1/LConn1
  PS-Simulink Converter1/LConn1 -- Voltage Sensor1/RConn1
  Switch/RConn1 -- Simulink-PS Converter/RConn1

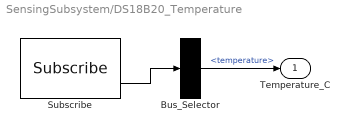
== system SensingSubsystem/DS18B20_Temperature ==
  Bus_Selector : BusSelector  OutputSignals=temperature
  Subscribe : ros2lib/Subscribe  topicSource=Specify your own  topic=/sandy/temperature  messageType=sensor_msgs/Temperature  sampleTime=0.1  QOSHistory=Keep last  QOSDepth=5  QOSReliability=Best effort  QOSDurability=Volatile  QOSDeadline=Inf  QOSLifespan=Inf  QOSLiveliness=Automatic  QOSLeaseDuration=Inf  QOSAvoidROSNamespaceConventions=off
  Temperature_C : Outport
  wires:
  Bus_Selector/1 -> Temperature_C/1  "<temperature>"
  Subscribe/2 -> Bus_Selector/1

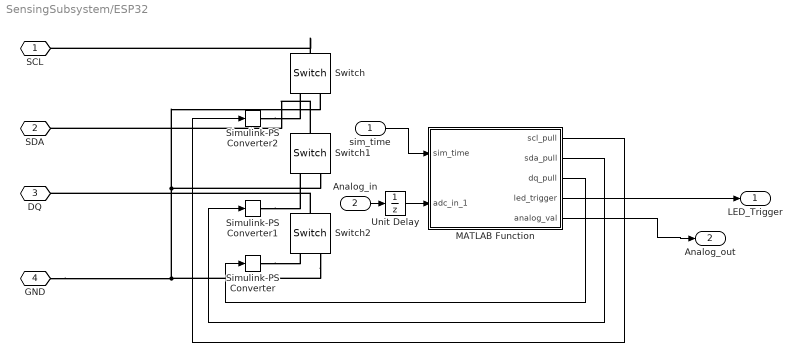
== system SensingSubsystem/ESP32 ==
  sim_time : Inport
  Analog_in : Inport  Port=2
  MATLAB Function : MATLAB Function  TreatAsAtomicUnit=on  SystemSampleTime=1e-3
  Simulink-PS Converter : nesl_utility/Simulink-PS Converter  PhysicalDomain=network_engine_domain  SubClassName=ps_input  LeftPortType=input  RightPortType=output  PseudoPeriodic=off  Frequencies=[]  NoiseDistribution=none  NoiseParameters=[]  Unit=1  AffineConversion=off  FilteringAndDerivatives=provide  SimscapeFilterOrder=1  InputFilterTimeConstant=0.001  UdotUserProvided=0
  Simulink-PS Converter1 : nesl_utility/Simulink-PS Converter  PhysicalDomain=network_engine_domain  SubClassName=ps_input  LeftPortType=input  RightPortType=output  PseudoPeriodic=off  Frequencies=[]  NoiseDistribution=none  NoiseParameters=[]  Unit=1  AffineConversion=off  FilteringAndDerivatives=provide  SimscapeFilterOrder=1  InputFilterTimeConstant=0.001  UdotUserProvided=0
  Simulink-PS Converter2 : nesl_utility/Simulink-PS Converter  PhysicalDomain=network_engine_domain  SubClassName=ps_input  LeftPortType=input  RightPortType=output  PseudoPeriodic=off  Frequencies=[]  NoiseDistribution=none  NoiseParameters=[]  Unit=1  AffineConversion=off  FilteringAndDerivatives=provide  SimscapeFilterOrder=1  InputFilterTimeConstant=0.001  UdotUserProvided=0
  Switch : fl_lib/Electrical/Electrical Elements/Switch  R_closed=0.01 Ohm  G_open=1e-8 1/Ohm  Threshold=0.5  i_specify=off  i_priority=None  i=0 A  i_nominal_specify=off  i_nominal_value=1  i_nominal_unit=A  v_specify=off  v_priority=None  v=0 V  v_nominal_specify=off  v_nominal_value=1  v_nominal_unit=V
  Switch1 : fl_lib/Electrical/Electrical Elements/Switch  R_closed=0.01 Ohm  G_open=1e-8 1/Ohm  Threshold=0.5  i_specify=off  i_priority=None  i=0 A  i_nominal_specify=off  i_nominal_value=1  i_nominal_unit=A  v_specify=off  v_priority=None  v=0 V  v_nominal_specify=off  v_nominal_value=1  v_nominal_unit=V
  Switch2 : fl_lib/Electrical/Electrical Elements/Switch  R_closed=0.01 Ohm  G_open=1e-8 1/Ohm  Threshold=0.5  i_specify=off  i_priority=None  i=0 A  i_nominal_specify=off  i_nominal_value=1  i_nominal_unit=A  v_specify=off  v_priority=None  v=0 V  v_nominal_specify=off  v_nominal_value=1  v_nominal_unit=V
  Unit Delay : UnitDelay  SampleTime=-1
  SCL : PMIOPort  Side=Left
  SDA : PMIOPort  Port=2  Side=Left
  DQ : PMIOPort  Port=3  Side=Left
  GND : PMIOPort  Port=4  Side=Left
  LED_Trigger : Outport
  Analog_out : Outport  Port=2
  wires:
  sim_time/1 -> MATLAB Function/1(sim_time)
  MATLAB Function/1(scl_pull) -> Simulink-PS Converter2/1
  MATLAB Function/2(sda_pull) -> Simulink-PS Converter1/1
  MATLAB Function/3(dq_pull) -> Simulink-PS Converter/1
  MATLAB Function/4(led_trigger) -> LED_Trigger/1
  MATLAB Function/5(analog_val) -> Analog_out/1
  Analog_in/1 -> Unit Delay/1
  Unit Delay/1 -> MATLAB Function/2(adc_in_1)
  connections:
  Switch/LConn1 -- SCL/RConn1
  Switch1/LConn1 -- SDA/RConn1
  Switch2/LConn1 -- DQ/RConn1
  GND/RConn1 -- Switch2/RConn2 -- Switch1/RConn2 -- Switch/RConn2
  Simulink-PS Converter/RConn1 -- Switch2/RConn1
  Simulink-PS Converter2/RConn1 -- Switch/RConn1
  Simulink-PS Converter1/RConn1 -- Switch1/RConn1

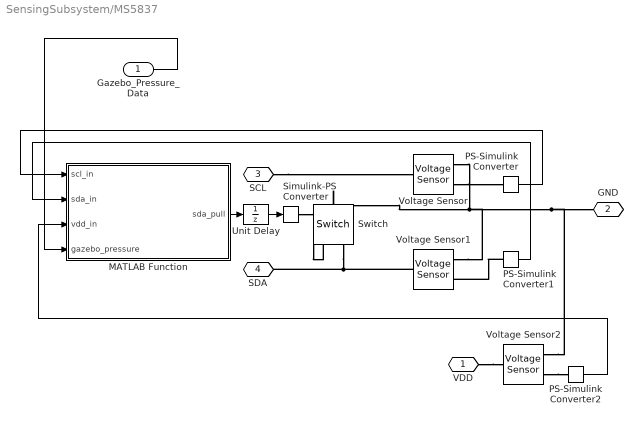
== system SensingSubsystem/MS5837 ==
  Gazebo_Pressure_Data : Inport
  MATLAB Function : MATLAB Function  TreatAsAtomicUnit=on  SystemSampleTime=1e-3
  PS-Simulink Converter : nesl_utility/PS-Simulink Converter  PhysicalDomain=network_engine_domain  SubClassName=ps_output  LeftPortType=input  RightPortType=output  PseudoPeriodic=off  Frequencies=[]  VectorFormat=inherit  Unit=inherit  AffineConversion=off
  PS-Simulink Converter1 : nesl_utility/PS-Simulink Converter  PhysicalDomain=network_engine_domain  SubClassName=ps_output  LeftPortType=input  RightPortType=output  PseudoPeriodic=off  Frequencies=[]  VectorFormat=inherit  Unit=inherit  AffineConversion=off
  PS-Simulink Converter2 : nesl_utility/PS-Simulink Converter  PhysicalDomain=network_engine_domain  SubClassName=ps_output  LeftPortType=input  RightPortType=output  PseudoPeriodic=off  Frequencies=[]  VectorFormat=inherit  Unit=inherit  AffineConversion=off
  Simulink-PS Converter : nesl_utility/Simulink-PS Converter  PhysicalDomain=network_engine_domain  SubClassName=ps_input  LeftPortType=input  RightPortType=output  PseudoPeriodic=off  Frequencies=[]  NoiseDistribution=none  NoiseParameters=[]  Unit=1  AffineConversion=off  FilteringAndDerivatives=provide  SimscapeFilterOrder=1  InputFilterTimeConstant=0.001  UdotUserProvided=0
  Switch : fl_lib/Electrical/Electrical Elements/Switch  R_closed=0.01 Ohm  G_open=1e-8 1/Ohm  Threshold=0.5  i_specify=off  i_priority=None  i=0 A  i_nominal_specify=off  i_nominal_value=1  i_nominal_unit=A  v_specify=off  v_priority=None  v=0 V  v_nominal_specify=off  v_nominal_value=1  v_nominal_unit=V
  Unit Delay : UnitDelay  SampleTime=-1
  Voltage Sensor : fl_lib/Electrical/Electrical Sensors/Voltage Sensor
  Voltage Sensor1 : fl_lib/Electrical/Electrical Sensors/Voltage Sensor
  Voltage Sensor2 : fl_lib/Electrical/Electrical Sensors/Voltage Sensor
  VDD : PMIOPort  Side=Left
  GND : PMIOPort  Port=2  Side=Left
  SCL : PMIOPort  Port=3  Side=Left
  SDA : PMIOPort  Port=4  Side=Left
  wires:
  PS-Simulink Converter1/1 -> MATLAB Function/2(sda_in)
  PS-Simulink Converter/1 -> MATLAB Function/1(scl_in)
  PS-Simulink Converter2/1 -> MATLAB Function/3(vdd_in)
  Gazebo_Pressure_Data/1 -> MATLAB Function/4(gazebo_pressure)
  MATLAB Function/1(sda_pull) -> Unit Delay/1
  Unit Delay/1 -> Simulink-PS Converter/1
  connections:
  SCL/RConn1 -- Voltage Sensor/LConn1
  Switch/LConn1 -- Voltage Sensor/RConn2 -- Voltage Sensor1/RConn2 -- GND/RConn1 -- Voltage Sensor2/RConn2
  Switch/RConn2 -- Voltage Sensor1/LConn1 -- SDA/RConn1
  Voltage Sensor/RConn1 -- PS-Simulink Converter/LConn1
  PS-Simulink Converter1/LConn1 -- Voltage Sensor1/RConn1
  Simulink-PS Converter/RConn1 -- Switch/RConn1
  VDD/RConn1 -- Voltage Sensor2/LConn1
  Voltage Sensor2/RConn1 -- PS-Simulink Converter2/LConn1

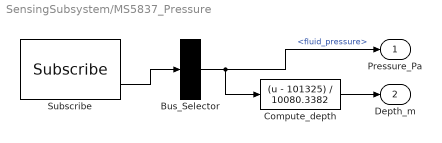
== system SensingSubsystem/MS5837_Pressure ==
  Bus_Selector : BusSelector  OutputSignals=fluid_pressure
  Compute_depth : Fcn  Expr=(u - 101325) / 10080.3382
  Subscribe : ros2lib/Subscribe  topicSource=Specify your own  topic=/sandy/pressure  messageType=sensor_msgs/FluidPressure  sampleTime=0.1  QOSHistory=Keep last  QOSDepth=5  QOSReliability=Best effort  QOSDurability=Volatile  QOSDeadline=Inf  QOSLifespan=Inf  QOSLiveliness=Automatic  QOSLeaseDuration=Inf  QOSAvoidROSNamespaceConventions=off
  Pressure_Pa : Outport
  Depth_m : Outport  Port=2
  wires:
  Compute_depth/1 -> Depth_m/1
  Bus_Selector/1 -> Compute_depth/1, Pressure_Pa/1  "<fluid_pressure>"
  Subscribe/2 -> Bus_Selector/1

== matlab function SensingSubsystem/DS18B20/MATLAB Function ==
  settings: updateMethod=DISCRETE
  data: dq_in input; vdd_in input; gazebo_temp input; dq_pull output
function dq_pull = onewire_slave_logic(dq_in, vdd_in, gazebo_temp)
    persistent state low_timer wait_timer bit_count current_byte bit_val prev_dq
    
    % Initialize variables
    if isempty(state)
        state = 1; 
        low_timer = 0; wait_timer = 0;
        bit_count = 0; current_byte = 0; bit_val = 0;
        prev_dq = 1;
    end
    
    dq_pull = 0; 
    
    % BROWNOUT PROTECTION
    if vdd_in < 3.0
        state = 1; low_timer = 0; return; 
    end
    
    % Edge detection for the ESP32's Read Time Slots
    dq_falling = (dq_in <= 0.5) && (prev_dq > 0.5);
    
    % 1-WIRE STATE MACHINE (1 loop = 1 microsecond)
    switch state
        case 1 % 'IDLE'
            if dq_in <= 0.5
                low_timer = low_timer + 1; 
            else
                if low_timer >= 480
                    state = 2; wait_timer = 0;
                end
                low_timer = 0; 
            end
            
        case 2 % 'WAIT_FOR_PRESENCE'
            wait_timer = wait_timer + 1;
            if wait_timer >= 30 
                state = 3; wait_timer = 0;
            end
            
        case 3 % 'SEND_PRESENCE'
            wait_timer = wait_timer + 1;
            if wait_timer <= 120
                dq_pull = 1; 
            else
                state = 4; % Move to WAIT_FOR_READ_SLOT
                bit_count = 1; % 1-Wire always sends the Least Significant Bit first!
                current_byte = gazebo_temp; 
            end
            
        case 4 % 'WAIT_FOR_READ_SLOT'
            % If the master pulls the line low, it wants a bit
            if dq_falling
                state = 5;
                wait_timer = 0;
                bit_val = double(bitget(uint8(current_byte), bit_count));
            end
            
        case 5 % 'SEND_BIT'
            wait_timer = wait_timer + 1;
            
            if bit_val == 0
                % Pull line low for 30us to send a '0'
                if wait_timer <= 30
                    dq_pull = 1;
                else
                    dq_pull = 0;
                end
            else
                % Do nothing (let it float high) to send a '1'
                dq_pull = 0; 
            end
            
            % Time slot ends after 60us, prepare for the next bit
            if wait_timer >= 60
                bit_count = bit_count + 1;
                if bit_count <= 8
                    state = 4; 
                else
                    state = 1; % Done sending byte, go to sleep
                end
            end
    end
    
    prev_dq = dq_in;
end

== matlab function SensingSubsystem/AS7341/MATLAB Function ==
  settings: updateMethod=DISCRETE
  data: scl_in input; sda_in input; vdd_in input; phyto_data input; sda_pull output
function sda_pull = i2c_slave_logic(scl_in, sda_in, vdd_in, phyto_data)
    %#codegen
    % I2C slave emulator for AS7341 (address 0x39).
    % Output: sda_pull. 1 = pull line low (open-drain ACK / data bit 0),
    %                   0 = release line (let pullup raise it to high).

    persistent state bit_count current_byte prev_scl prev_sda

    % State encoding:
    %   1 = IDLE
    %   2 = READ_ADDRESS
    %   3 = WAIT_ACK_FALL
    %   4 = HOLD_ACK
    %   5 = SEND_DATA
    %   6 = WAIT_MASTER_NACK

    if isempty(state)
        state         = uint8(1);
        bit_count     = uint8(0);
        current_byte  = uint8(0);
        prev_scl      = 1.0;
        prev_sda      = 1.0;
    end

    sda_pull = 0;

    % Brownout: reset to IDLE if VDD too low.
    if vdd_in < 1.8
        state = uint8(1);
        prev_scl = scl_in;
        prev_sda = sda_in;
        return;
    end

    % Edge detection.
    scl_rising  = (scl_in  >  0.5) && (prev_scl <= 0.5);
    scl_falling = (scl_in  <= 0.5) && (prev_scl >  0.5);
    sda_falling = (sda_in  <= 0.5) && (prev_sda >  0.5);

    switch state
        case 1  % IDLE — wait for START condition (SDA falls while SCL high)
            if sda_falling && (scl_in > 0.5)
                state        = uint8(2);
                bit_count    = uint8(0);
                current_byte = uint8(0);
            end

        case 2  % READ_ADDRESS — shift in 7 address bits + 1 R/W bit
            if scl_rising
                current_byte = bitshift(current_byte, 1);
                if sda_in > 0.5
                    current_byte = current_byte + uint8(1);
                end
                bit_count = bit_count + uint8(1);

                if bit_count == uint8(8)
                    address = bitshift(current_byte, -1);
                    if address == uint8(57)   % 0x39 = AS7341
                        state = uint8(3);
                    else
                        state = uint8(1);
                    end
                end
            end

        case 3  % WAIT_ACK_FALL — let 8th clock pulse finish before ACKing
            if scl_falling
                state = uint8(4);
            end

        case 4  % HOLD_ACK — pull SDA low to acknowledge
            sda_pull = 1;
            if scl_falling
                state        = uint8(5);
                bit_count    = uint8(8);
                current_byte = uint8(phyto_data(1));
            end

        case 5  % SEND_DATA — shift out 8 data bits, MSB first
            if bit_count > uint8(0)
                bit_val = bitget(current_byte, bit_count);
                if bit_val == uint8(1)
                    sda_pull = 0;   % Release line (open-drain high)
                else
                    sda_pull = 1;   % Pull line low
                end
                if scl_falling
                    bit_count = bit_count - uint8(1);
                    if bit_count == uint8(0)
                        state = uint8(6);
                    end
                end
            end

        case 6  % WAIT_MASTER_NACK — give bus back to master
            sda_pull = 0;
            if scl_falling
                state = uint8(1);
            end

        otherwise
            state = uint8(1);
    end

    prev_scl = scl_in;
    prev_sda = sda_in;
end

== matlab function SensingSubsystem/MS5837/MATLAB Function ==
  settings: updateMethod=DISCRETE
  data: scl_in input; sda_in input; vdd_in input; gazebo_pressure input; sda_pull output
function sda_pull = ms5837_slave_logic(scl_in, sda_in, vdd_in, gazebo_pressure)
    persistent state bit_count current_byte prev_scl prev_sda
    
    if isempty(state)
        state = 1; bit_count = 0; current_byte = 0;
        prev_scl = 1; prev_sda = 1;
    end
    
    sda_pull = 0;
    if vdd_in < 1.5, state = 1; return; end

    % Edge Detection
    scl_rising  = (scl_in > 0.5)  && (prev_scl <= 0.5);
    scl_falling = (scl_in <= 0.5) && (prev_scl > 0.5);
    sda_falling = (sda_in <= 0.5) && (prev_sda > 0.5);

    switch state
        case 1 % IDLE
            if sda_falling && (scl_in > 0.5)
                state = 2; bit_count = 0; current_byte = 0;
            end
        case 2 % READ_ADDRESS
            if scl_rising
                current_byte = bitshift(current_byte, 1);
                if sda_in > 0.5, current_byte = current_byte + 1; end
                bit_count = bit_count + 1;
                if bit_count == 8
                    if bitshift(current_byte, -1) == hex2dec('76')
                        state = 3; 
                    else
                        state = 1;
                    end
                end
            end
        case 3 % WAIT_ACK_FALL
            if scl_falling, state = 4; end
        case 4 % HOLD_ACK
            sda_pull = 1;
            if scl_falling
                state = 5; bit_count = 8;
                current_byte = gazebo_pressure; 
            end
        case 5 % SEND_DATA (The missing part!)
            if bit_count > 0
                bit_val = double(bitget(uint8(current_byte), bit_count));
                sda_pull = double(bit_val == 0);                if scl_falling
                    bit_count = bit_count - 1;
                    if bit_count == 0, state = 6; end
                end
            end
        case 6 % WAIT_NACK
            if scl_falling, state = 1; end
    end
    prev_scl = scl_in; prev_sda = sda_in;
end

== matlab function SensingSubsystem/ESP32/MATLAB Function ==
  settings: updateMethod=DISCRETE
  data: scl_pull output; sim_time input; sda_pull output; dq_pull output; adc_in_1 input; led_trigger output; analog_val output
function [scl_pull, sda_pull, dq_pull, led_trigger, analog_val] = esp32_master(sim_time, adc_in_1)
% Persistent variable to store the result of the ADC conversion
persistent saved_adc
if isempty(saved_adc)
    saved_adc = 0;
end

% Default Initialization: All switches open (float high) and LED off
scl_pull = 0; 
sda_pull = 0; 
dq_pull = 0; 
led_trigger = 0;

% --- WINDOW 1: 1-WIRE TEMPERATURE (0.5s - 0.6s) ---
if sim_time >= 0.5000 && sim_time < 0.6000
    % DS18B20 Reset Pulse (500 microseconds)
    if sim_time < 0.5005
        dq_pull = 1;
        % DS18B20 Read Time Slots (8 bits)
    elseif sim_time >= 0.5010 && sim_time < 0.5018
        t_1w = sim_time - 0.5010;
        if mod(t_1w, 0.000100) < 0.000005
            dq_pull = 1; % Tiny 5us trigger pulse for each bit
        end
    end

    % --- I2C INITIALIZATION (0.6s - 1.0s) ---
elseif sim_time >= 0.6000 && sim_time < 1.0000
    sda_pull = 1; % I2C START Condition
    if sim_time >= 0.6001
        scl_pull = 1;
    end

    % --- WINDOW 2 & 3: I2C SENSORS (1.0s - 1.4s) ---
elseif sim_time >= 1.0000 && sim_time < 1.4000
    period = 0.000010; % 100kHz
    half_period = period / 2;

    if sim_time < 1.2000
        % SESSION 1: Light Sensor (0x39)
        t_session = sim_time - 1.0000;
        target_addr = [1, 0, 0, 0, 1, 1, 0, 1]; % 0x39 Address (Inverted)
    else
        % SESSION 2: Pressure Sensor (0x76)
        t_session = sim_time - 1.2000;
        target_addr = [0, 0, 0, 1, 0, 0, 1, 1]; % 0x76 Address (Inverted)
    end

    % START CONDITION: Pull SDA down 1us before SCL
    if t_session == 0
        sda_pull = 1; 
        scl_pull = 0;
    elseif t_session > 0 && t_session < (period * 18)
        % Clock generation (using double() to avoid Coder type errors)
        scl_pull = double(mod(t_session, period) < half_period);
        % Data generation
        cycle_num = floor(t_session / period) + 1;
        if cycle_num <= 8
            sda_pull = target_addr(cycle_num);
        else
            sda_pull = 0; % Release for ACK/Data phase
        end
    end

    % --- WINDOW 4: ANALOG SENSING (1.4s - 1.5s) ---
elseif sim_time >= 1.4000 && sim_time < 1.5000
    % Pulse the high-power Blue LED to excite the phytoplankton
    led_trigger = 1; 

    % Sample the ADC voltage (0V to 3.3V) 
    % Convert to 12-bit integer (0 to 4095) for the final data reading
    if sim_time >= 1.4000 && sim_time < 1.4001
        % We "snap" the photo here to avoid noise
        saved_adc = (adc_in_1 / 3.3) * 4095;
    end
end

% Final output is the persistent digital value of the last light sample
analog_val = saved_adc;
end

== matlab function SensingSubsystem/BPW34_Photodiode/Reduce_to_scalar ==
  data: msg input Bus: SL_Bus_sensor_msgs_Image; I output
function I = reduce_bpw34(msg)
    %#codegen
    
    % Extract the relevant data field from the ROS message bus.
    % Replace '.data' with '.illuminance' or your custom field name if different.
    I = double(msg.data); 
end
